simulink model "states"  (R2020b)
settings: Solver=FixedStepDiscrete  StartTime=0.0  StopTime=60.0  FixedStep=0.1  RelTol=1e-3  EnableMultiTasking=on
settings Model: Creator=ana  LastModifiedBy=ana
settings SolverCC: AutoInsertRateTranBlk=on
settings OptimizationCC: LifeSpan=inf
settings DebuggingCC: SFUnexpectedBacktrackingDiag=warning  SFNoUnconditionalDefaultTransitionDiag=warning  SFExecutionAtInitializationDiag=none  ArithmeticOperatorsInVariantConditions=warning
settings SFSimCC: SimUseLocalCustomCode=off  CustomCodeUndefinedFunction=UseInterfaceOnly
settings RTWCC: RTWUseLocalCustomCode=off
settings CodeAppCC: StateflowObjectComments=on
settings GRTTargetCC: TargetLangStandard=C89/C90 (ANSI)
settings ConfigComp: CovMetricSettings=dw  CovSaveCumulativeToWorkspaceVar=on  CovSaveSingleToWorkspaceVar=on  CovExternalEMLEnable=off

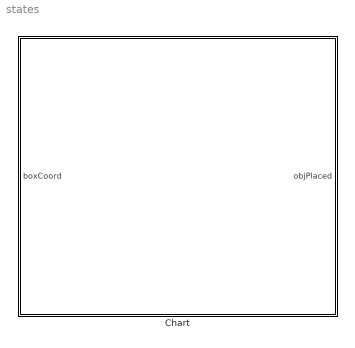
== system states ==
  Chart : Stateflow chart  TreatAsAtomicUnit=on

== stateflow chart states/Chart ==
  state HomePosition
    entry:
    % robot coordinates as input from environment
    % periodically check if there are any objects to be picked up
  state DetectObject
    % detect object with sensors and pass on coordinates
    [objDetected, objCoord] = SensorDetection();
  state Execute
    entry:
    stopConveyor();
    objPicked = false;
    objPlaced = false;
    state Pick
      state ComputeGraspPose
        % at the top of the object
        graspCoord = GraspPose(objCoord);
      state MoveToReachPosition
        % move from current home
        % position to the grasp pose
        send(grabCoord, Dynamic)
      state PickUpObject
        % activate gripper
      state MoveToRetractedPosition
        % move from grasp pose to
        % retracted position
        exit:
        objPicked = true;
      (default) -> ComputeGraspPose
      ComputeGraspPose -> MoveToReachPosition
      PickUpObject -> Execute.Pick.MoveToRetractedPosition
      MoveToReachPosition -> PickUpObject
    state Place
      state ComputePlacementPosition
        % call placement algorithm to
        % get position
        placeCoord = PlacementAlgorithm(objCoord, boxCoord);
      state MoveToRetractedPosition
        % move from current placement
        % position to the retracted pose
        exit:
        objPlaced = true;
      state MoveToPlacementPosition
        % move from current retracted
        % position to the placement pose
        send(placeCoord, Dynamic)
      state PlaceObject
        % deactivate gripper
      (default) -> ComputePlacementPosition
      ComputePlacementPosition -> MoveToPlacementPosition
      PlaceObject -> Execute.Place.MoveToRetractedPosition
      MoveToPlacementPosition -> PlaceObject
    (default) -> Pick
    Pick -> Place : [objPicked]
  (default) -> HomePosition
  HomePosition -> DetectObject : after(1, sec)
  Place -> HomePosition : [objPlaced]
  DetectObject -> HomePosition [order 2] : [~objDetected]
  DetectObject -> Execute [order 1] : [objDetected]
  data: boxCoord input; objPicked local; objDetected local; placeCoord local; objCoord local; graspCoord local; objPlaced output; grabCoord local
  events: stopConveyor local FUNCTION_CALL_EVENT
  function SensorDetection:
    | function SensorDetection
  function GraspPose:
    | function GraspPose
  function PlacementAlgorithm:
    | function PlacementAlgorithm
